simulink model "manning_3test_nonlinear"  (R2022b)
settings: Solver=VariableStepAuto  StartTime=0.0  StopTime=5*N  RelTol=1e-3
libraries: cstblocks x1
settings Model: Creator=chuan  LastModifiedBy=chuan

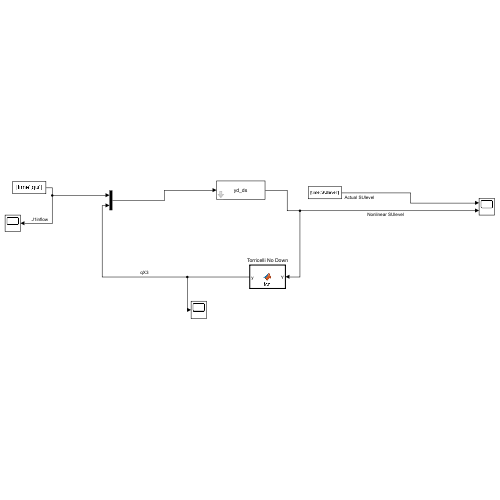
[thumbnail: Simulink's stored preview of the top-level diagram]
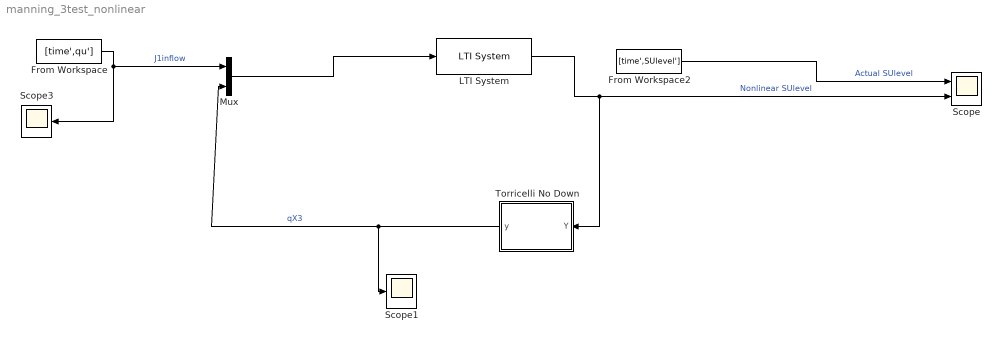
== system manning_3test_nonlinear ==
  From Workspace : FromWorkspace  VariableName=[time',qu']
  From Workspace2 : FromWorkspace  VariableName=[time',SUlevel']
  LTI System : cstblocks/LTI System  sys=yd_ds  IC=[]
  Mux : Mux  Inputs=2
  Scope : Scope  NumInputPorts=2
  Scope1 : Scope
  Scope3 : Scope
  Torricelli No Down : MATLAB Function  TreatAsAtomicUnit=on
  wires:
  LTI System/1 -> Torricelli No Down/1(Y), Scope/2  "Nonlinear SUlevel"
  Mux/1 -> LTI System/1
  From Workspace/1 -> Mux/1, Scope3/1  "J1inflow"
  Torricelli No Down/1(y) -> Scope1/1, Mux/2  "qX3"
  From Workspace2/1 -> Scope/1  "Actual SUlevel"

== matlab function manning_3test_nonlinear/Torricelli No Down ==
  data: Y input; y output
function y = fcn(Y)
Cd = 0.65;
A0 = 100;
g = 9.81;
Z0 = 3;
Yfull = 10;
H_star = Z0 + Yfull;

Y = max(Y,0);
H1 = Y + Z0;

if H1 >= H_star
    He = H1 - (Z0 + Yfull/2);
    y = Cd*A0*sqrt(2*g*He);
else
    CwL = (Cd*A0*sqrt(g))/(Yfull);
    y = CwL*(H1-Z0)^(1.5);
end
